simulink model "Unit_Test_Debug_Control"  (R2018b)
settings: Solver=FixedStepDiscrete  StartTime=0.0  StopTime=10.0  FixedStep=fswParams.sample_time_s  RelTol=1e-3
undefined symbols (not defined in the file): fswParams, Mekf_joseph, Mekf_joseph_Lib
libraries: aerolibutil x6, sharedutil x4, dspmtrx3 x2, extended_kalman_filter_lib x1, MEKF_lib x1, satelliteDynamics_lib x1
settings Model: Creator=kashton6  LastModifiedBy=kashton6
settings DataIOCC: ReturnWorkspaceOutputs=on

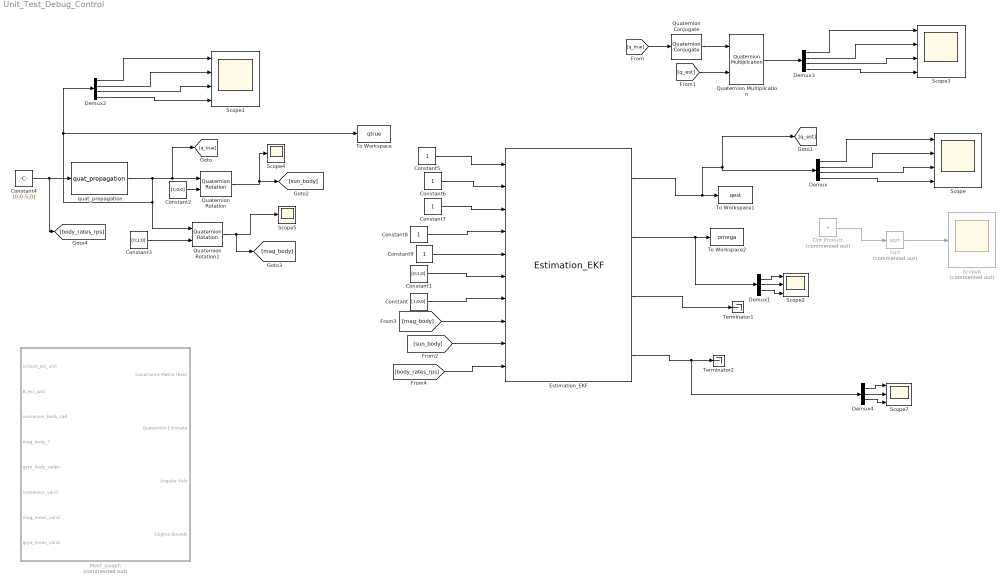
== system Unit_Test_Debug_Control ==
  Constant : Constant  Value=[1;0;0]  VectorParams1D=off
  Constant1 : Constant  Value=[0;1;0]  VectorParams1D=off
  Constant2 : Constant  Value=[1;0;0]  VectorParams1D=off
  Constant3 : Constant  Value=[0;1;0]  VectorParams1D=off
  Constant4 : Constant  Value=[0;0.5;0]  VectorParams1D=off
  Constant{5..9} (5 alike) : Constant
  Demux : Demux
  Demux1 : Demux  Outputs=3
  Demux2 : Demux
  Demux3 : Demux
  Demux4 : Demux  Outputs=3
  Dot Product : DotProduct  Commented=on  InputSameDT=on  OutDataTypeStr=Inherit: Inherit via internal rule
  "Estimation_EKF " : extended_kalman_filter_lib/Estimation_EKF   SystemSampleTime=-1
      link override " ": InitialCondition=fswParams.ekf.ic.rt_valid_gyro
      link override " 1": InitialCondition=fswParams.ekf.ic.rt_valid_mag
      link override " 10": InitialCondition=fswParams.ekf.ic.rt_meas_cov
      link override " 11": InitialCondition=fswParams.ekf.ic.rt_sun_eci_est
      link override " 2": InitialCondition=fswParams.ekf.ic.rt_valid_sun
      link override " 3": InitialCondition=fswParams.ekf.ic.rt_w_body_radps
      link override " 4": InitialCondition=fswParams.ekf.ic.rt_mag_body
      link override " 5": InitialCondition=fswParams.ekf.ic.rt_mag_eci_est
      link override " 6": InitialCondition=fswParams.ekf.ic.rt_sun_body
      link override " 7": InitialCondition=fswParams.ekf.ic.rt_mt_power_ok
      link override " 8": InitialCondition=fswParams.ekf.ic.rt_sc_in_sun
      link override Constant1: Value=fswParams.ekf.meas_cov
      link override Propagate Step /Constant3: Value=fswParams.ekf.proc_cov
      link override Propagate Step /G: Value=fswParams.ekf.G
  Mekf_joseph : Subsystem  Commented=on  AncestorBlock=Mekf_joseph/Mekf_joseph_Lib
  Quaternion Conjugate : aerolibutil/Quaternion Conjugate
      settings: SourceProductName=Aerospace Blockset  SourceProductBaseCode=AE
  Quaternion Multiplication : aerolibutil/Quaternion Multiplication
  Quaternion Rotation : aerolibutil/Quaternion Rotation
  Quaternion Rotation1 : aerolibutil/Quaternion Rotation
  Scope : Scope  NumInputPorts=4
  Scope1 : Scope  NumInputPorts=4
  Scope2 : Scope  NumInputPorts=3
  Scope3 : Scope  NumInputPorts=4
  Scope4 : Scope
  Scope5 : Scope
  Scope6 : Scope  Commented=on
  Scope7 : Scope  NumInputPorts=3
  Sqrt : Sqrt  Commented=on  SaturateOnIntegerOverflow=on
  Terminator1 : Terminator
  Terminator2 : Terminator
  To Workspace : ToWorkspace  VariableName=qtrue  SaveFormat=Timeseries  SampleTime=-1
  To Workspace1 : ToWorkspace  VariableName=qest  SaveFormat=Timeseries  SampleTime=-1
  To Workspace2 : ToWorkspace  VariableName=omega  SaveFormat=Timeseries  SampleTime=-1
  quat_propagation : satelliteDynamics_lib/satelliteDynamics_lib/quat_propagation  SystemSampleTime=-1
  wires:
  Demux3/4 -> Scope3/4
  Sqrt/1 -> Scope6/1
  [q_est] -> Quaternion Multiplication/2
  Dot Product/1 -> Sqrt/1
  Demux3/3 -> Scope3/3
  Demux2/4 -> Scope1/4
  Quaternion Rotation1/1 -> [mag_body], Scope5/1
  Demux3/2 -> Scope3/2
  [q_true] -> Quaternion Conjugate/1
  Demux2/1 -> Scope1/1
  Constant3/1 -> Quaternion Rotation1/2
  Quaternion Multiplication/1 -> Demux3/1
  quat_propagation/1 -> Demux2/1, To Workspace/1, Quaternion Rotation1/1, [q_true], Quaternion Rotation/1
  Demux2/3 -> Scope1/3
  Constant4/1 -> [body_rates_rps], quat_propagation/1
  Constant2/1 -> Quaternion Rotation/2
  Demux1/1 -> Scope2/1
  Demux1/2 -> Scope2/2
  Demux1/3 -> Scope2/3
  Demux3/1 -> Scope3/1
  Demux/3 -> Scope/3
  Quaternion Rotation/1 -> [sun_body], Scope4/1
  Demux/4 -> Scope/4
  Demux/2 -> Scope/2
  Demux/1 -> Scope/1
  Quaternion Conjugate/1 -> Quaternion Multiplication/1
  Demux2/2 -> Scope1/2
  Constant/1 -> "Estimation_EKF "/7
  Constant1/1 -> "Estimation_EKF "/6
  [sun_body] -> "Estimation_EKF "/9
  [mag_body] -> "Estimation_EKF "/8
  [body_rates_rps] -> "Estimation_EKF "/10
  Constant5/1 -> "Estimation_EKF "/1
  Constant6/1 -> "Estimation_EKF "/2
  Constant7/1 -> "Estimation_EKF "/3
  Constant8/1 -> "Estimation_EKF "/4
  Constant9/1 -> "Estimation_EKF "/5
  "Estimation_EKF "/1 -> [q_est], Demux/1, To Workspace1/1
  "Estimation_EKF "/2 -> Demux1/1, To Workspace2/1
  "Estimation_EKF "/3 -> Terminator1/1
  Demux4/3 -> Scope7/3
  "Estimation_EKF "/4 -> Demux4/1, Terminator2/1
  Demux4/2 -> Scope7/2
  Demux4/1 -> Scope7/1

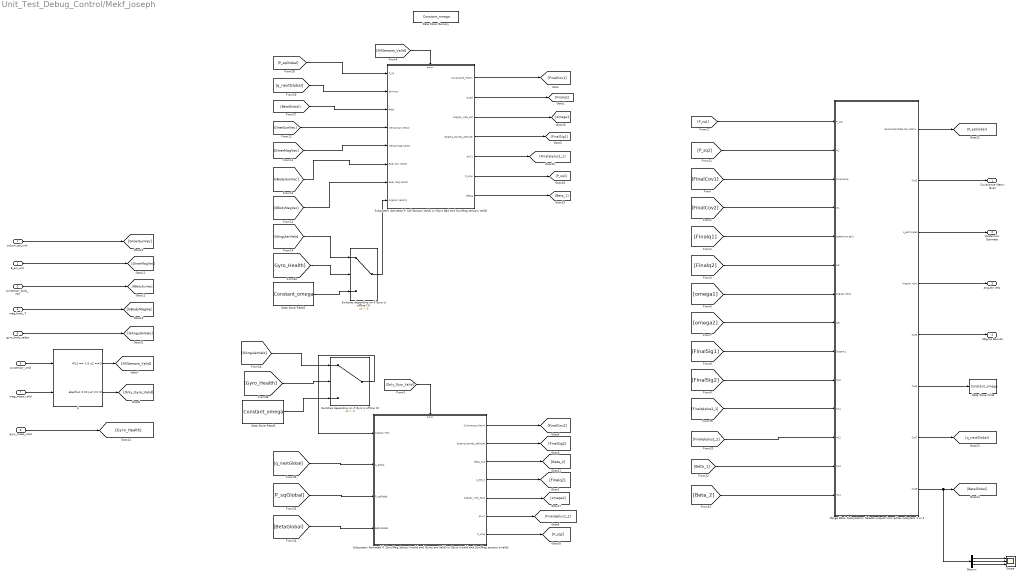
== system Unit_Test_Debug_Control/Mekf_joseph ==
  sc2sun_eci_unit : Inport
  B_eci_unit : Inport  Port=2
  sunsensor_body_rad : Inport  Port=3
  mag_body_T : Inport  Port=4
  gyro_body_radps : Inport  Port=5
  sunsensor_valid : Inport  Port=6
  mag_meas_valid : Inport  Port=7
  gryo_meas_valid : Inport  Port=8
  Data Store Memory : DataStoreMemory  DataStoreName=Constant_omega  ReadBeforeWriteMsg=warning  WriteAfterWriteMsg=warning  WriteAfterReadMsg=warning  InitialValue=fswParams.estimation.ic.w_init  VectorParams1D=off  ShowAdditionalParam=off
  Data Store Read2 : DataStoreRead  DataStoreName=Constant_omega
  Data Store Read3 : DataStoreRead  DataStoreName=Constant_omega
  Data Store Write : DataStoreWrite  DataStoreName=Constant_omega
  Demux : Demux  Outputs=3
  If : If  NumInputs=2  IfExpression=u1 == 1 & u2 ==1  ElseIfExpressions=u1 ==0 |u2 == 0  ShowElse=off
  "Merge Block Subsystems, Selects outputs from either subsytem 1 or 2" : Subsystem
  Scope : Scope  NumInputPorts=3
  Subsystem Activated if: [All Sensors Valid] or [Gyro Bad and Sun/Mag sensors Valid] : Subsystem  TreatAsAtomicUnit=on
  Subsystem Activated if: [Sun/Mag Sensor Invalid and Gyros are Valid] or [Gyro Invalid and Sun/Mag sensors Invalid] : Subsystem  TreatAsAtomicUnit=on
  Switches depending on if Gyro is offline (1) : Switch  Criteria=u2 > Threshold
  Switches depending on if Gyro is offline (2) : Switch  Criteria=u2 > Threshold
  Covariance Matrix (6x6) : Outport
  "Quaternion Estimate " : Outport  Port=2
  "Angular Velo " : Outport  Port=3
  "3Sigma Bounds " : Outport  Port=4
  wires:
  Subsystem Activated if: [Sun/Mag Sensor Invalid and Gyros are Valid] or [Gyro Invalid and Sun/Mag sensors Invalid]/6(qk+1) -> [Finalqkplus1_2]
  Switches depending on if Gyro is offline (2)/1 -> Subsystem Activated if: [Sun/Mag Sensor Invalid and Gyros are Valid] or [Gyro Invalid and Sun/Mag sensors Invalid]/1(Angular Velo)
  Switches depending on if Gyro is offline (1)/1 -> Subsystem Activated if: [All Sensors Valid] or [Gyro Bad and Sun/Mag sensors Valid]/8(Angular Velocity)
  [GAngularVelo] -> Switches depending on if Gyro is offline (1)/1
  [GAngularVelo] -> Switches depending on if Gyro is offline (2)/1
  [GBodySunVec] -> Subsystem Activated if: [All Sensors Valid] or [Gyro Bad and Sun/Mag sensors Valid]/6(Body Sun Vector)
  [GInerMagVec] -> Subsystem Activated if: [All Sensors Valid] or [Gyro Bad and Sun/Mag sensors Valid]/5(Inertial Mag Vector)
  [GBodyMagVec] -> Subsystem Activated if: [All Sensors Valid] or [Gyro Bad and Sun/Mag sensors Valid]/7(Body Mag Vector)
  Subsystem Activated if: [All Sensors Valid] or [Gyro Bad and Sun/Mag sensors Valid]/2(q_est) -> [Finalq1]
  Subsystem Activated if: [All Sensors Valid] or [Gyro Bad and Sun/Mag sensors Valid]/1(Covariance_Matrix) -> [FinalCov1]
  [Only_Gyro_Valid] -> Subsystem Activated if: [Sun/Mag Sensor Invalid and Gyros are Valid] or [Gyro Invalid and Sun/Mag sensors Invalid]/Action
  Subsystem Activated if: [All Sensors Valid] or [Gyro Bad and Sun/Mag sensors Valid]/4(3sigma_bounds_attitude) -> [FinalSig1]
  Subsystem Activated if: [Sun/Mag Sensor Invalid and Gyros are Valid] or [Gyro Invalid and Sun/Mag sensors Invalid]/4(q_est_k) -> [Finalq2]
  [GInerSunVec] -> Subsystem Activated if: [All Sensors Valid] or [Gyro Bad and Sun/Mag sensors Valid]/4(Inertial Sun Vector)
  Subsystem Activated if: [Sun/Mag Sensor Invalid and Gyros are Valid] or [Gyro Invalid and Sun/Mag sensors Invalid]/1(Covariance_Matrix) -> [FinalCov2]
  [AllSensors_Valid] -> Subsystem Activated if: [All Sensors Valid] or [Gyro Bad and Sun/Mag sensors Valid]/Action
  Subsystem Activated if: [Sun/Mag Sensor Invalid and Gyros are Valid] or [Gyro Invalid and Sun/Mag sensors Invalid]/2(3sigma_bounds_attitude) -> [FinalSig2]
  [q_nextGlobal] -> Subsystem Activated if: [Sun/Mag Sensor Invalid and Gyros are Valid] or [Gyro Invalid and Sun/Mag sensors Invalid]/2(q_global)
  Subsystem Activated if: [All Sensors Valid] or [Gyro Bad and Sun/Mag sensors Valid]/5(qk+1) -> [Finalqkplus1_1]
  [P_sqGlobal] -> Subsystem Activated if: [Sun/Mag Sensor Invalid and Gyros are Valid] or [Gyro Invalid and Sun/Mag sensors Invalid]/3(P_sqGlobal)
  [BetaGlobal] -> Subsystem Activated if: [Sun/Mag Sensor Invalid and Gyros are Valid] or [Gyro Invalid and Sun/Mag sensors Invalid]/4(Beta Global)
  [BetaGlobal] -> Subsystem Activated if: [All Sensors Valid] or [Gyro Bad and Sun/Mag sensors Valid]/3(Beta)
  Subsystem Activated if: [All Sensors Valid] or [Gyro Bad and Sun/Mag sensors Valid]/3(Angular_Velo_est) -> [omega1]
  Subsystem Activated if: [All Sensors Valid] or [Gyro Bad and Sun/Mag sensors Valid]/6("P_prop ") -> [P_sq1]
  Subsystem Activated if: [All Sensors Valid] or [Gyro Bad and Sun/Mag sensors Valid]/7(Betaa) -> [Beta_1]
  Subsystem Activated if: [Sun/Mag Sensor Invalid and Gyros are Valid] or [Gyro Invalid and Sun/Mag sensors Invalid]/7("P_prop ") -> [P_sq2]
  Subsystem Activated if: [Sun/Mag Sensor Invalid and Gyros are Valid] or [Gyro Invalid and Sun/Mag sensors Invalid]/3(Beta_Out) -> [Beta_2]
  Subsystem Activated if: [Sun/Mag Sensor Invalid and Gyros are Valid] or [Gyro Invalid and Sun/Mag sensors Invalid]/5(Angular_Velo_est1) -> [omega2]
  [q_nextGlobal] -> Subsystem Activated if: [All Sensors Valid] or [Gyro Bad and Sun/Mag sensors Valid]/2(qkminus)
  [P_sqGlobal] -> Subsystem Activated if: [All Sensors Valid] or [Gyro Bad and Sun/Mag sensors Valid]/1(P_sq)
  If/1 -> [AllSensors_Valid]
  If/2 -> [Only_Gyro_Valid]
  [Gyro_Health] -> Switches depending on if Gyro is offline (1)/2
  Data Store Read2/1 -> Switches depending on if Gyro is offline (1)/3
  [Gyro_Health] -> Switches depending on if Gyro is offline (2)/2
  Data Store Read3/1 -> Switches depending on if Gyro is offline (2)/3
  [P_sq1] -> "Merge Block Subsystems, Selects outputs from either subsytem 1 or 2"/1(P_sq1)
  [P_sq2] -> "Merge Block Subsystems, Selects outputs from either subsytem 1 or 2"/2(In2)
  [FinalCov1] -> "Merge Block Subsystems, Selects outputs from either subsytem 1 or 2"/3(covariance)
  [FinalCov2] -> "Merge Block Subsystems, Selects outputs from either subsytem 1 or 2"/4(In4)
  [Finalq1] -> "Merge Block Subsystems, Selects outputs from either subsytem 1 or 2"/5(quaternion est1)
  [Finalq2] -> "Merge Block Subsystems, Selects outputs from either subsytem 1 or 2"/6(In6)
  [omega1] -> "Merge Block Subsystems, Selects outputs from either subsytem 1 or 2"/7(angular velo1)
  [omega2] -> "Merge Block Subsystems, Selects outputs from either subsytem 1 or 2"/8(In8)
  [FinalSig1] -> "Merge Block Subsystems, Selects outputs from either subsytem 1 or 2"/9(3sigma 1)
  [FinalSig2] -> "Merge Block Subsystems, Selects outputs from either subsytem 1 or 2"/10(In10)
  [Finalqkplus1_1] -> "Merge Block Subsystems, Selects outputs from either subsytem 1 or 2"/11(In11)
  [Finalqkplus1_2] -> "Merge Block Subsystems, Selects outputs from either subsytem 1 or 2"/12(In12)
  [Beta_1] -> "Merge Block Subsystems, Selects outputs from either subsytem 1 or 2"/13(In13)
  [Beta_2] -> "Merge Block Subsystems, Selects outputs from either subsytem 1 or 2"/14(In14)
  "Merge Block Subsystems, Selects outputs from either subsytem 1 or 2"/1(Squre Root State Cov Matrix) -> [P_sqGlobal]
  "Merge Block Subsystems, Selects outputs from either subsytem 1 or 2"/2(Out2) -> Covariance Matrix (6x6)/1
  "Merge Block Subsystems, Selects outputs from either subsytem 1 or 2"/3(q_estimated) -> "Quaternion Estimate "/1
  "Merge Block Subsystems, Selects outputs from either subsytem 1 or 2"/4(Angular Velo) -> "Angular Velo "/1
  "Merge Block Subsystems, Selects outputs from either subsytem 1 or 2"/6(Out5) -> Data Store Write/1
  "Merge Block Subsystems, Selects outputs from either subsytem 1 or 2"/5(Out6) -> "3Sigma Bounds "/1
  "Merge Block Subsystems, Selects outputs from either subsytem 1 or 2"/7(Out7) -> [q_nextGlobal]
  sc2sun_eci_unit/1 -> [GInerSunVec]
  sunsensor_body_rad/1 -> [GBodySunVec]
  sunsensor_valid/1 -> If/1
  mag_meas_valid/1 -> If/2
  gryo_meas_valid/1 -> [Gyro_Health]
  B_eci_unit/1 -> [GInerMagVec]
  mag_body_T/1 -> [GBodyMagVec]
  gyro_body_radps/1 -> [GAngularVelo]
  Demux/3 -> Scope/3
  Demux/2 -> Scope/2
  "Merge Block Subsystems, Selects outputs from either subsytem 1 or 2"/8(Out8) -> Demux/1, [BetaGlobal]
  Demux/1 -> Scope/1

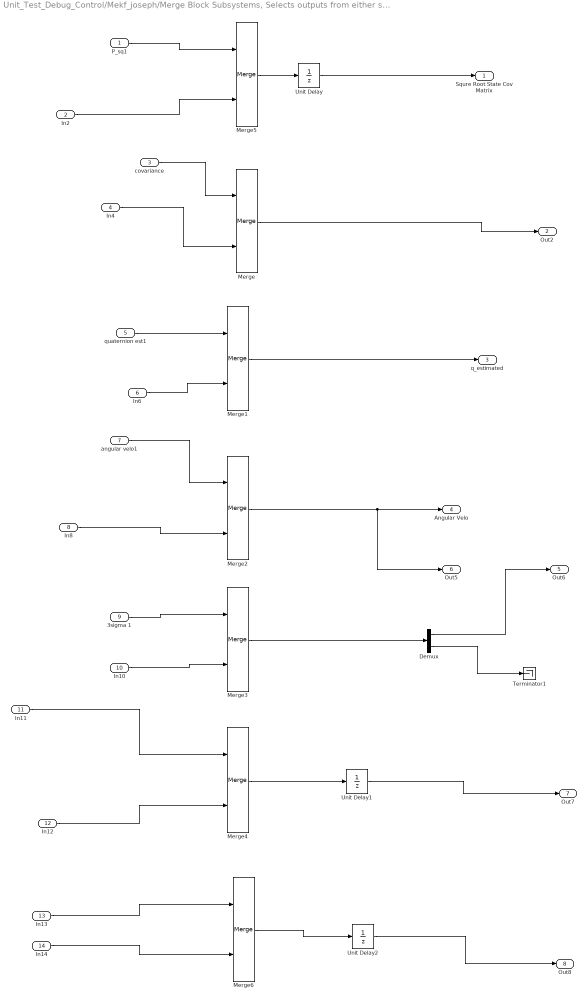
== system Unit_Test_Debug_Control/Mekf_joseph/Merge Block Subsystems, Selects outputs from either subsytem 1 or 2 ==
  P_sq1 : Inport
  In2 : Inport  Port=2
  covariance : Inport  Port=3
  In4 : Inport  Port=4
  quaternion est1 : Inport  Port=5
  In6 : Inport  Port=6
  angular velo1 : Inport  Port=7
  In8 : Inport  Port=8
  3sigma 1 : Inport  Port=9
  In10 : Inport  Port=10
  In11 : Inport  Port=11
  In12 : Inport  Port=12
  In13 : Inport  Port=13
  In14 : Inport  Port=14
  Demux : Demux  Outputs=2
  Merge{,1..6} (7 alike) : Merge
  Terminator1 : Terminator
  Unit Delay : UnitDelay  InitialCondition=fswParams.estimation.ic.P_init  SampleTime=-1  HasFrameUpgradeWarning=on
  Unit Delay1 : UnitDelay  InitialCondition=fswParams.estimation.ic.quat_est_init  SampleTime=-1  HasFrameUpgradeWarning=on
  Unit Delay2 : UnitDelay  InitialCondition=fswParams.estimation.ic.Beta_init  SampleTime=-1  HasFrameUpgradeWarning=on
  Squre Root State Cov Matrix : Outport
  Out2 : Outport  Port=2
  q_estimated : Outport  Port=3
  Angular Velo : Outport  Port=4
  Out6 : Outport  Port=5
  Out5 : Outport  Port=6
  Out7 : Outport  Port=7
  Out8 : Outport  Port=8
  wires:
  Merge3/1 -> Demux/1
  Merge2/1 -> Out5/1, Angular Velo/1
  Unit Delay1/1 -> Out7/1
  Demux/2 -> Terminator1/1
  Merge6/1 -> Unit Delay2/1
  3sigma 1/1 -> Merge3/1
  quaternion est1/1 -> Merge1/1
  In14/1 -> Merge6/2
  angular velo1/1 -> Merge2/1
  In11/1 -> Merge4/1
  Merge5/1 -> Unit Delay/1
  In10/1 -> Merge3/2
  In2/1 -> Merge5/2
  covariance/1 -> Merge/1
  Merge4/1 -> Unit Delay1/1
  In4/1 -> Merge/2
  Demux/1 -> Out6/1
  In13/1 -> Merge6/1
  Merge/1 -> Out2/1
  In6/1 -> Merge1/2
  In8/1 -> Merge2/2
  In12/1 -> Merge4/2
  P_sq1/1 -> Merge5/1
  Unit Delay2/1 -> Out8/1
  Unit Delay/1 -> Squre Root State Cov Matrix/1
  Merge1/1 -> q_estimated/1

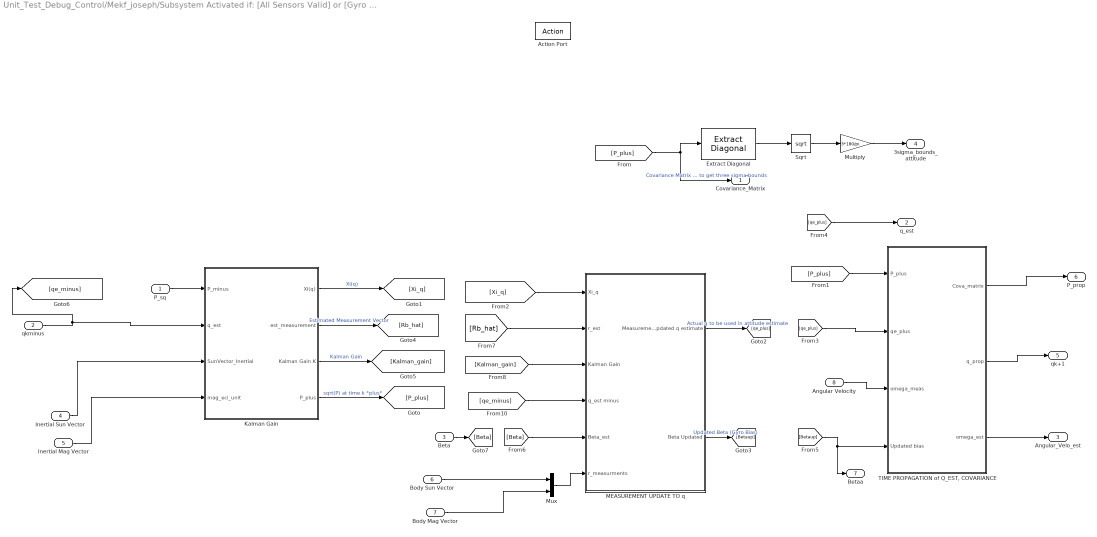
== system Unit_Test_Debug_Control/Mekf_joseph/Subsystem Activated if: [All Sensors Valid] or [Gyro Bad and Sun//Mag sensors Valid] ==
  P_sq : Inport
  qkminus : Inport  Port=2
  Beta : Inport  Port=3
  Inertial Sun Vector : Inport  Port=4
  Inertial Mag Vector : Inport  Port=5
  Body Sun Vector : Inport  Port=6
  Body Mag Vector : Inport  Port=7
  Angular Velocity : Inport  Port=8
  Action Port : ActionPort
  Extract Diagonal : dspmtrx3/Extract Diagonal
      settings: SourceProductName=DSP System Toolbox  SourceProductBaseCode=DS
  Kalman Gain : Subsystem  AncestorBlock=MEKF_LibraryR2018b/Multiplicative Extended Kalman Filter/Kalman Gain
  "MEASUREMENT UPDATE TO q " : Subsystem  AncestorBlock=MEKF_LibraryR2018b/Multiplicative Extended Kalman Filter/MEASUREMENT UPDATE TO q AND COVARIANCE2
  Multiply : Gain  Gain=3*180/pi
  Mux : Mux  Inputs=2
  Sqrt : Sqrt  SaturateOnIntegerOverflow=on
  "TIME PROPAGATION of Q_EST, COVARIANCE" : Subsystem  AncestorBlock=MEKF_Library/Multiplicative Extended Kalman Filter/TIME PROPAGATION of Q_EST, COVARIANCE
  Covariance_Matrix : Outport
  q_est : Outport  Port=2
  Angular_Velo_est : Outport  Port=3
  3sigma_bounds_attitude : Outport  Port=4
  qk+1 : Outport  Port=5
  "P_prop " : Outport  Port=6
  Betaa : Outport  Port=7
  wires:
  Inertial Sun Vector/1 -> Kalman Gain/3(SunVector_Inertial)
  [qe_plus] -> q_est/1
  "TIME PROPAGATION of Q_EST, COVARIANCE"/2(q_prop) -> qk+1/1
  "TIME PROPAGATION of Q_EST, COVARIANCE"/3(omega_est) -> Angular_Velo_est/1
  [P_plus] -> Extract Diagonal/1, Covariance_Matrix/1  "Covariance Matrix from which to get three sigma bounds"
  qkminus/1 -> [qe_minus], Kalman Gain/2(q_est)
  Extract Diagonal/1 -> Sqrt/1
  Angular Velocity/1 -> "TIME PROPAGATION of Q_EST, COVARIANCE"/3(omega_meas)
  P_sq/1 -> Kalman Gain/1(P_minus)
  [qe_plus] -> "TIME PROPAGATION of Q_EST, COVARIANCE"/2(qe_plus)
  "MEASUREMENT UPDATE TO q "/2(Beta Updated) -> [Betaup]  "Updated Beta (Gyro Bias)"
  [Rb_hat] -> "MEASUREMENT UPDATE TO q "/2(r_est)
  "TIME PROPAGATION of Q_EST, COVARIANCE"/1(Cova_matrix) -> "P_prop "/1
  Kalman Gain/4(P_plus) -> [P_plus]  "sqrt(P) at time k *plus*"
  Kalman Gain/3(Kalman Gain K) -> [Kalman_gain]  "Kalman Gain"
  [qe_minus] -> "MEASUREMENT UPDATE TO q "/4(q_est minus)
  Kalman Gain/1(Xi(q)) -> [Xi_q]  "Xi(q)"
  Sqrt/1 -> Multiply/1
  [Betaup] -> "TIME PROPAGATION of Q_EST, COVARIANCE"/4(Updated bias), Betaa/1
  [Beta] -> "MEASUREMENT UPDATE TO q "/5(Beta_est)
  "MEASUREMENT UPDATE TO q "/1(Measurement updated q estimate) -> [qe_plus]  "Actual q to be used in attitude estimate"
  [P_plus] -> "TIME PROPAGATION of Q_EST, COVARIANCE"/1(P_plus)
  Kalman Gain/2(est_measurement) -> [Rb_hat]  "Estimated Measurement Vector"
  [Xi_q] -> "MEASUREMENT UPDATE TO q "/1(Xi_q)
  [Kalman_gain] -> "MEASUREMENT UPDATE TO q "/3(Kalman Gain)
  Inertial Mag Vector/1 -> Kalman Gain/4("mag_eci_unit ")
  Body Sun Vector/1 -> Mux/1
  Body Mag Vector/1 -> Mux/2
  Mux/1 -> "MEASUREMENT UPDATE TO q "/6(r_measurments)
  Multiply/1 -> 3sigma_bounds_attitude/1
  Beta/1 -> [Beta]

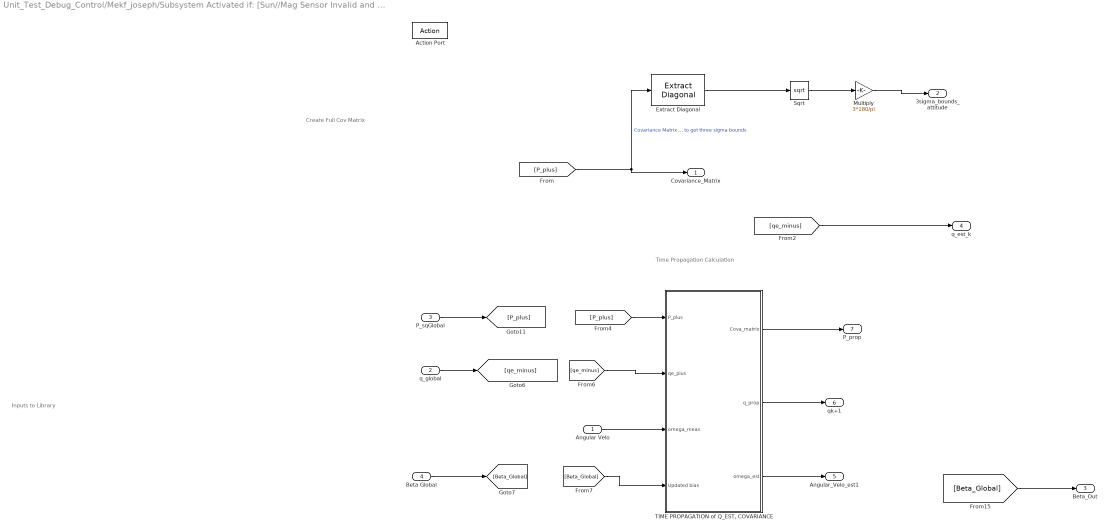
== system Unit_Test_Debug_Control/Mekf_joseph/Subsystem Activated if: [Sun//Mag Sensor Invalid and Gyros are Valid] or [Gyro Invalid and Sun//Mag sensors Invalid] ==
  note: Time Propagation Calculation
  note: Inputs to Library
  note: Create Full Cov Matrix
  Angular Velo : Inport
  q_global : Inport  Port=2
  P_sqGlobal : Inport  Port=3
  Beta Global : Inport  Port=4
  Action Port : ActionPort
  Extract Diagonal : dspmtrx3/Extract Diagonal
      settings: SourceProductName=DSP System Toolbox  SourceProductBaseCode=DS
  Multiply : Gain  Gain=3*180/pi
  Sqrt : Sqrt  SaturateOnIntegerOverflow=on
  "TIME PROPAGATION of Q_EST, COVARIANCE" : Subsystem  AncestorBlock=|
      | Mekf_joseph/Mekf_joseph_Lib/Subsystem Activated if: [All Sensors Valid]
      | or
      | [Gyro Bad and Sun//Mag sensors Valid]/TIME PROPAGATION of Q_EST, COVARIANCE
  Covariance_Matrix : Outport
  3sigma_bounds_attitude : Outport  Port=2
  Beta_Out : Outport  Port=3
  q_est_k : Outport  Port=4
  Angular_Velo_est1 : Outport  Port=5
  qk+1 : Outport  Port=6
  "P_prop " : Outport  Port=7
  wires:
  [P_plus] -> "TIME PROPAGATION of Q_EST, COVARIANCE"/1(P_plus)
  "TIME PROPAGATION of Q_EST, COVARIANCE"/2(q_prop) -> qk+1/1
  "TIME PROPAGATION of Q_EST, COVARIANCE"/1(Cova_matrix) -> "P_prop "/1
  [Beta_Global] -> "TIME PROPAGATION of Q_EST, COVARIANCE"/4(Updated bias)
  "TIME PROPAGATION of Q_EST, COVARIANCE"/3(omega_est) -> Angular_Velo_est1/1
  Angular Velo/1 -> "TIME PROPAGATION of Q_EST, COVARIANCE"/3(omega_meas)
  [qe_minus] -> "TIME PROPAGATION of Q_EST, COVARIANCE"/2(qe_plus)
  q_global/1 -> [qe_minus]
  Beta Global/1 -> [Beta_Global]
  Extract Diagonal/1 -> Sqrt/1
  P_sqGlobal/1 -> [P_plus]
  [qe_minus] -> q_est_k/1
  [P_plus] -> Extract Diagonal/1, Covariance_Matrix/1  "Covariance Matrix from which to get three sigma bounds"
  [Beta_Global] -> Beta_Out/1
  Multiply/1 -> 3sigma_bounds_attitude/1
  Sqrt/1 -> Multiply/1

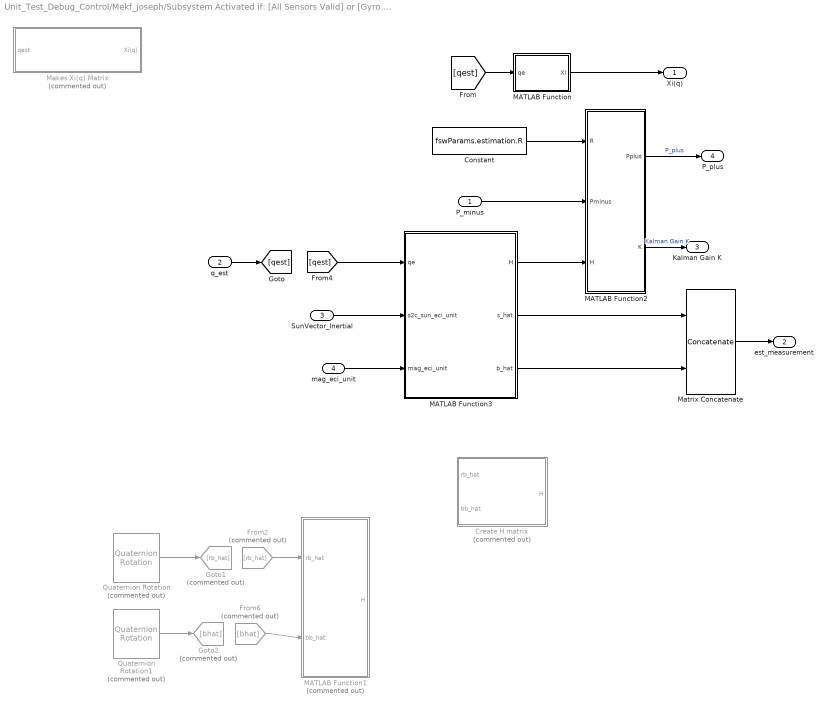
== system Unit_Test_Debug_Control/Mekf_joseph/Subsystem Activated if: [All Sensors Valid] or [Gyro Bad and Sun//Mag sensors Valid]/Kalman Gain ==
  P_minus : Inport
  q_est : Inport  Port=2
  SunVector_Inertial : Inport  Port=3
  "mag_eci_unit " : Inport  Port=4
  Constant : Constant  Value=fswParams.estimation.R  VectorParams1D=off
  Create H matrix : Subsystem  Commented=on
  From2 : From  Commented=on  GotoTag=rb_hat
  From6 : From  Commented=on  GotoTag=bhat
  Goto1 : Goto  Commented=on  GotoTag=rb_hat
  Goto2 : Goto  Commented=on  GotoTag=bhat
  MATLAB Function : MATLAB Function  TreatAsAtomicUnit=on
  MATLAB Function1 : MATLAB Function  Commented=on  TreatAsAtomicUnit=on
  MATLAB Function2 : MATLAB Function  TreatAsAtomicUnit=on
  MATLAB Function3 : MATLAB Function  TreatAsAtomicUnit=on
  Makes Xi(q) Matrix : Subsystem  Commented=on
  Matrix Concatenate : Concatenate  Mode=Multidimensional array
  Quaternion Rotation : aerolibutil/Quaternion Rotation  Commented=on
  Quaternion Rotation1 : aerolibutil/Quaternion Rotation  Commented=on
  Xi(q) : Outport
  est_measurement : Outport  Port=2
  Kalman Gain K : Outport  Port=3
  P_plus : Outport  Port=4
  wires:
  MATLAB Function3/1(H) -> MATLAB Function2/3(H)
  "mag_eci_unit "/1 -> MATLAB Function3/3(mag_eci_unit)
  SunVector_Inertial/1 -> MATLAB Function3/2(s2c_sun_eci_unit)
  [qest] -> MATLAB Function3/1(qe)
  From6/1 -> MATLAB Function1/2(bb_hat)
  From2/1 -> MATLAB Function1/1(rb_hat)
  P_minus/1 -> MATLAB Function2/2(Pminus)
  MATLAB Function2/2(K) -> Kalman Gain K/1  "Kalman Gain K"
  MATLAB Function2/1(Pplus) -> P_plus/1  "P_plus"
  q_est/1 -> [qest]
  Quaternion Rotation/1 -> Goto1/1
  Quaternion Rotation1/1 -> Goto2/1
  MATLAB Function3/2(s_hat) -> Matrix Concatenate/1
  MATLAB Function3/3(b_hat) -> Matrix Concatenate/2
  Matrix Concatenate/1 -> est_measurement/1
  Constant/1 -> MATLAB Function2/1(R)
  [qest] -> MATLAB Function/1(qe)
  MATLAB Function/1(XI) -> Xi(q)/1

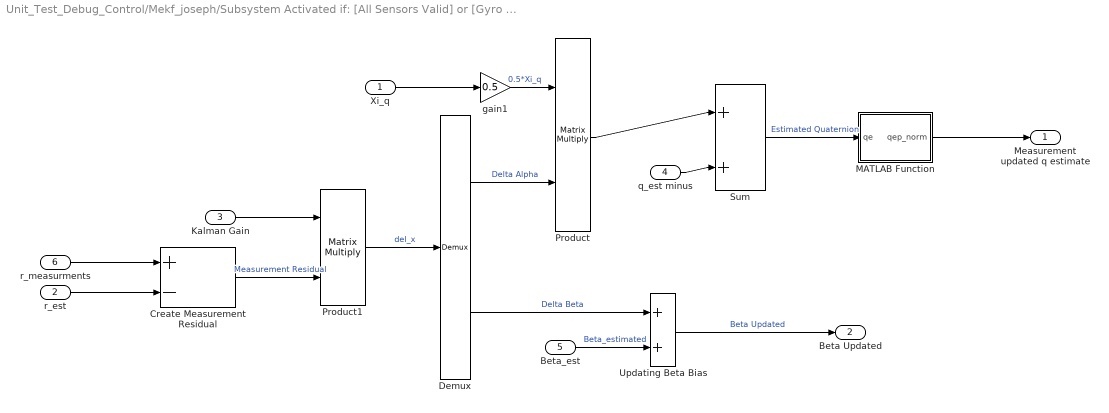
== system Unit_Test_Debug_Control/Mekf_joseph/Subsystem Activated if: [All Sensors Valid] or [Gyro Bad and Sun//Mag sensors Valid]/MEASUREMENT UPDATE TO q  ==
  Xi_q : Inport
  r_est : Inport  Port=2
  Kalman Gain : Inport  Port=3
  q_est minus : Inport  Port=4
  Beta_est : Inport  Port=5
  r_measurments : Inport  Port=6
  Create Measurement Residual : Sum  Inputs=+-
  Demux : Demux  Outputs=[3;3]
  MATLAB Function : MATLAB Function  TreatAsAtomicUnit=on
  Product : Product  Inputs=**  Multiplication=Matrix(*)
  Product1 : Product  Multiplication=Matrix(*)
  Sum : Sum  Inputs=|++
  "Updating Beta Bias " : Sum
  gain1 : Gain  Gain=0.5
  Measurement updated q estimate : Outport
  Beta Updated : Outport  Port=2
  wires:
  Demux/1 -> Product/2  "Delta Alpha"
  gain1/1 -> Product/1  "0.5*Xi_q"
  Demux/2 -> "Updating Beta Bias "/1  "Delta Beta"
  Product/1 -> Sum/1
  Product1/1 -> Demux/1  "del_x"
  r_est/1 -> Create Measurement Residual/2
  Create Measurement Residual/1 -> Product1/2  "Measurement Residual"
  "Updating Beta Bias "/1 -> Beta Updated/1  "Beta Updated"
  Beta_est/1 -> "Updating Beta Bias "/2  "Beta_estimated"
  q_est minus/1 -> Sum/2
  Kalman Gain/1 -> Product1/1
  r_measurments/1 -> Create Measurement Residual/1
  Xi_q/1 -> gain1/1
  Sum/1 -> MATLAB Function/1(qe)  "Estimated Quaternion"
  MATLAB Function/1(qep_norm) -> Measurement updated q estimate/1

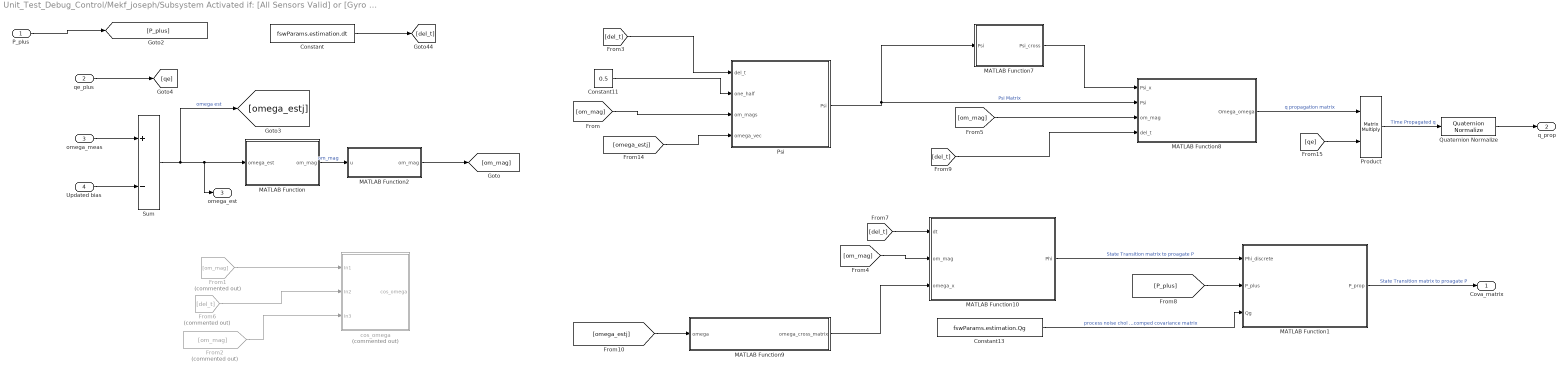
== system Unit_Test_Debug_Control/Mekf_joseph/Subsystem Activated if: [All Sensors Valid] or [Gyro Bad and Sun//Mag sensors Valid]/TIME PROPAGATION of Q_EST, COVARIANCE ==
  P_plus : Inport
  qe_plus : Inport  Port=2
  omega_meas : Inport  Port=3
  Updated bias : Inport  Port=4
  Constant : Constant  Value=fswParams.estimation.dt
  Constant11 : Constant  Value=0.5
  Constant13 : Constant  Value=fswParams.estimation.Qg  VectorParams1D=off
  From1 : From  Commented=on  GotoTag=om_mag
  From2 : From  Commented=on  GotoTag=om_mag
  From6 : From  Commented=on  GotoTag=del_t
  MATLAB Function : MATLAB Function  TreatAsAtomicUnit=on
  MATLAB Function1 : MATLAB Function  TreatAsAtomicUnit=on
  MATLAB Function10 : MATLAB Function  TreatAsAtomicUnit=on
  MATLAB Function2 : MATLAB Function  TreatAsAtomicUnit=on
  MATLAB Function7 : MATLAB Function  TreatAsAtomicUnit=on
  MATLAB Function8 : MATLAB Function  TreatAsAtomicUnit=on
  MATLAB Function9 : MATLAB Function  TreatAsAtomicUnit=on
  Product : Product  Multiplication=Matrix(*)
  Psi : Subsystem
  Quaternion Normalize : sharedutil/Quaternion Normalize  aMode=aMode
      settings: SourceProductName=Aerospace Blockset  SourceProductBaseCode=AE
  Sum : Sum  Inputs=+-
  cos_omega : Subsystem  Commented=on
  Cova_matrix : Outport
  q_prop : Outport  Port=2
  omega_est : Outport  Port=3
  wires:
  Quaternion Normalize/1 -> q_prop/1
  P_plus/1 -> [P_plus]
  qe_plus/1 -> [qe]
  Updated bias/1 -> Sum/2
  omega_meas/1 -> Sum/1
  [del_t] -> MATLAB Function8/4(del_t)
  MATLAB Function7/1(Psi_cross) -> MATLAB Function8/1(Psi_x)
  MATLAB Function8/1(Omega_omega) -> Product/1  "q propagation matrix"
  MATLAB Function9/1(omega_cross_matrix) -> MATLAB Function10/3(omega_x)
  MATLAB Function10/1(Phi) -> MATLAB Function1/1(Phi_discrete)  "State Transition matrix to proagate P"
  Product/1 -> Quaternion Normalize/1  "Time Propagated q"
  Constant13/1 -> MATLAB Function1/3(Qg)  "process noise chol decomped covariance matrix"
  MATLAB Function/1(om_mag) -> MATLAB Function2/1(u)  "om_mag"
  [om_mag] -> MATLAB Function10/2(om_mag)
  [om_mag] -> MATLAB Function8/3(om_mag)
  [del_t] -> MATLAB Function10/1(dt)
  [P_plus] -> MATLAB Function1/2(P_plus)
  [omega_estj] -> MATLAB Function9/1(omega)
  [qe] -> Product/2
  From1/1 -> cos_omega/1(In1)
  From2/1 -> cos_omega/3(In3)
  Psi/1(Psi) -> MATLAB Function8/2(Psi), MATLAB Function7/1(Psi)  "Psi Matrix"
  [del_t] -> Psi/1(del_t)
  Constant11/1 -> Psi/2(one_half)
  [omega_estj] -> Psi/4(omega_vec)
  [om_mag] -> Psi/3(om_mags)
  Sum/1 -> MATLAB Function/1(omega_est), omega_est/1, [omega_estj]  "omega est"
  From6/1 -> cos_omega/2(In2)
  Constant/1 -> [del_t]
  MATLAB Function2/1(om_mag) -> [om_mag]
  MATLAB Function1/1(P_prop) -> Cova_matrix/1  "State Transition matrix to proagate P"

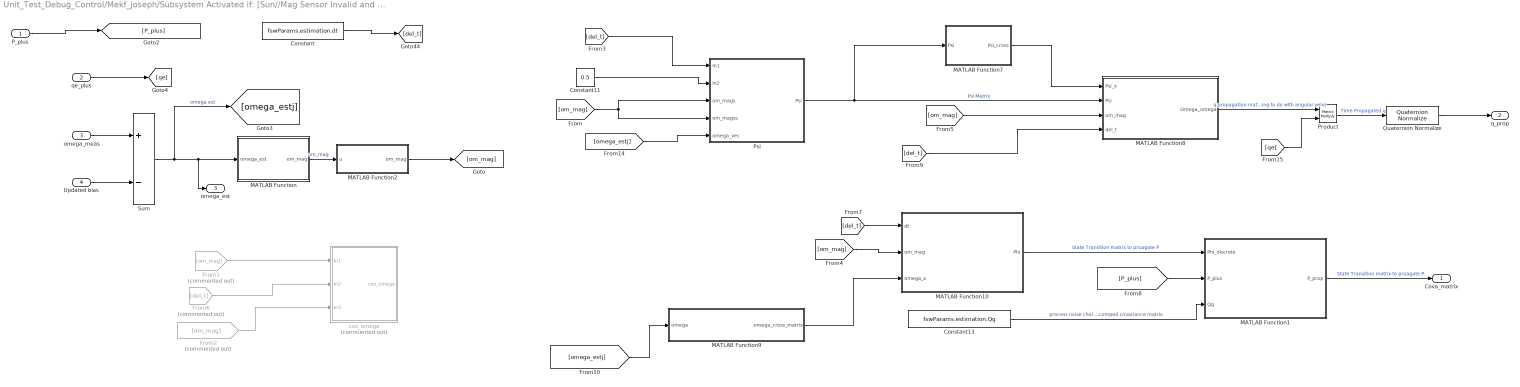
== system Unit_Test_Debug_Control/Mekf_joseph/Subsystem Activated if: [Sun//Mag Sensor Invalid and Gyros are Valid] or [Gyro Invalid and Sun//Mag sensors Invalid]/TIME PROPAGATION of Q_EST, COVARIANCE ==
  P_plus : Inport
  qe_plus : Inport  Port=2
  omega_meas : Inport  Port=3
  Updated bias : Inport  Port=4
  Constant : Constant  Value=fswParams.estimation.dt
  Constant11 : Constant  Value=0.5
  Constant13 : Constant  Value=fswParams.estimation.Qg  VectorParams1D=off
  From1 : From  Commented=on  GotoTag=om_mag
  From2 : From  Commented=on  GotoTag=om_mag
  From6 : From  Commented=on  GotoTag=del_t
  MATLAB Function : MATLAB Function  TreatAsAtomicUnit=on
  MATLAB Function1 : MATLAB Function  TreatAsAtomicUnit=on
  MATLAB Function10 : MATLAB Function  TreatAsAtomicUnit=on
  MATLAB Function2 : MATLAB Function  TreatAsAtomicUnit=on
  MATLAB Function7 : MATLAB Function  TreatAsAtomicUnit=on
  MATLAB Function8 : MATLAB Function  TreatAsAtomicUnit=on
  MATLAB Function9 : MATLAB Function  TreatAsAtomicUnit=on
  Product : Product  Multiplication=Matrix(*)
  Psi : Subsystem
  Quaternion Normalize : sharedutil/Quaternion Normalize  aMode=aMode
      settings: SourceProductName=Aerospace Blockset  SourceProductBaseCode=AE
  Sum : Sum  Inputs=+-
  cos_omega : Subsystem  Commented=on
  Cova_matrix : Outport
  q_prop : Outport  Port=2
  omega_est : Outport  Port=3
  wires:
  Quaternion Normalize/1 -> q_prop/1
  P_plus/1 -> [P_plus]
  qe_plus/1 -> [qe]
  Updated bias/1 -> Sum/2
  omega_meas/1 -> Sum/1
  [del_t] -> MATLAB Function8/4(del_t)
  MATLAB Function7/1(Psi_cross) -> MATLAB Function8/1(Psi_x)
  MATLAB Function8/1(Omega_omega) -> Product/1  "q propagation matrix (nothing to do with angular velo)"
  MATLAB Function9/1(omega_cross_matrix) -> MATLAB Function10/3(omega_x)
  MATLAB Function10/1(Phi) -> MATLAB Function1/1(Phi_discrete)  "State Transition matrix to proagate P"
  Product/1 -> Quaternion Normalize/1  "Time Propagated q"
  Constant13/1 -> MATLAB Function1/3(Qg)  "process noise chol decomped covariance matrix"
  MATLAB Function/1(om_mag) -> MATLAB Function2/1(u)  "om_mag"
  [om_mag] -> MATLAB Function10/2(om_mag)
  [om_mag] -> MATLAB Function8/3(om_mag)
  [del_t] -> MATLAB Function10/1(dt)
  [P_plus] -> MATLAB Function1/2(P_plus)
  [omega_estj] -> MATLAB Function9/1(omega)
  [qe] -> Product/2
  From1/1 -> cos_omega/1(In1)
  From2/1 -> cos_omega/3(In3)
  Psi/1(Psi) -> MATLAB Function8/2(Psi), MATLAB Function7/1(Psi)  "Psi Matrix"
  [del_t] -> Psi/1(In1)
  Constant11/1 -> Psi/2(In2)
  [omega_estj] -> Psi/5(omega_vec)
  [om_mag] -> Psi/3(om_mags), Psi/4(om_magss)
  Sum/1 -> MATLAB Function/1(omega_est), omega_est/1, [omega_estj]  "omega est"
  From6/1 -> cos_omega/2(In2)
  Constant/1 -> [del_t]
  MATLAB Function2/1(om_mag) -> [om_mag]
  MATLAB Function1/1(P_prop) -> Cova_matrix/1  "State Transition matrix to proagate P"

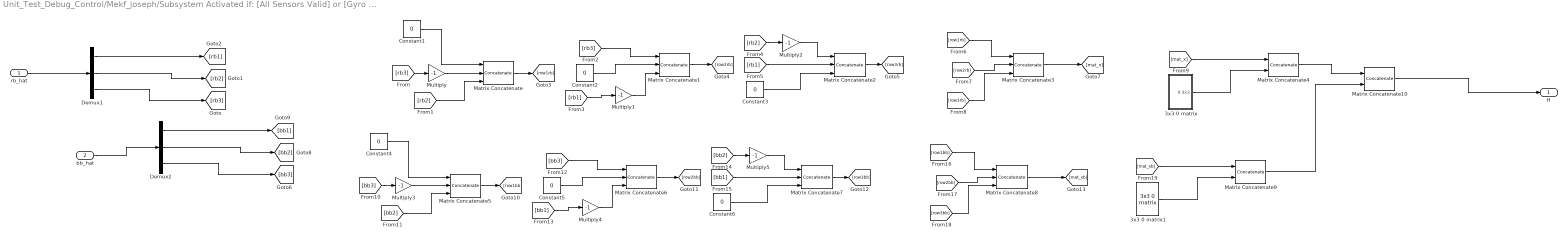
== system Unit_Test_Debug_Control/Mekf_joseph/Subsystem Activated if: [All Sensors Valid] or [Gyro Bad and Sun//Mag sensors Valid]/Kalman Gain/Create H matrix ==
  rb_hat : Inport
  bb_hat : Inport  Port=2
  3x3 0 matrix : Subsystem
  3x3 0 matrix1 : MEKF_lib/MEKF_lib/Subsystem Activated if: [All Sensors Valid] or [Gyro Bad and Sun//Mag sensors Valid]/Kalman Gain/Create H matrix/3x3 0 matrix  SystemSampleTime=-1
  Constant{1..6} (6 alike) : Constant  Value=0
  Demux1 : Demux  Outputs=3
  Demux2 : Demux  Outputs=3
  Matrix Concatenate{,1..2,5..7} (6 alike) : Concatenate  NumInputs=3  Mode=Multidimensional array  ConcatenateDimension=2
  Matrix Concatenate10 : Concatenate  Mode=Multidimensional array
  Matrix Concatenate3 : Concatenate  NumInputs=3  Mode=Multidimensional array
  Matrix Concatenate4 : Concatenate  Mode=Multidimensional array  ConcatenateDimension=2
  Matrix Concatenate8 : Concatenate  NumInputs=3  Mode=Multidimensional array
  Matrix Concatenate9 : Concatenate  Mode=Multidimensional array  ConcatenateDimension=2
  Multiply{,1..5} (6 alike) : Gain  Gain=-1
  H : Outport
  wires:
  Matrix Concatenate1/1 -> [row2rb]
  Multiply/1 -> Matrix Concatenate/2
  [mat_x] -> Matrix Concatenate4/1
  Demux1/2 -> [rb2]
  Multiply2/1 -> Matrix Concatenate2/1
  [row3rb] -> Matrix Concatenate3/3
  Matrix Concatenate/1 -> [row1rb]
  Matrix Concatenate2/1 -> [row3rb]
  [rb1] -> Multiply1/1
  [rb3] -> Multiply/1
  Multiply1/1 -> Matrix Concatenate1/3
  Constant3/1 -> Matrix Concatenate2/3
  3x3 0 matrix/1(0 3x3) -> Matrix Concatenate4/2
  [rb2] -> Multiply2/1
  [rb2] -> Matrix Concatenate/3
  [rb3] -> Matrix Concatenate1/1
  [row2rb] -> Matrix Concatenate3/2
  Constant1/1 -> Matrix Concatenate/1
  [row1rb] -> Matrix Concatenate3/1
  Demux1/1 -> [rb1]
  Matrix Concatenate3/1 -> [mat_x]
  Constant2/1 -> Matrix Concatenate1/2
  [rb1] -> Matrix Concatenate2/2
  Demux1/3 -> [rb3]
  rb_hat/1 -> Demux1/1
  Demux2/3 -> [bb3]
  bb_hat/1 -> Demux2/1
  Demux2/1 -> [bb1]
  Demux2/2 -> [bb2]
  Multiply5/1 -> Matrix Concatenate7/1
  [bb1] -> Matrix Concatenate7/2
  Constant4/1 -> Matrix Concatenate5/1
  Multiply3/1 -> Matrix Concatenate5/2
  Constant5/1 -> Matrix Concatenate6/2
  Multiply4/1 -> Matrix Concatenate6/3
  Matrix Concatenate5/1 -> [row1bb]
  [bb1] -> Multiply4/1
  Matrix Concatenate7/1 -> [row3bb]
  Constant6/1 -> Matrix Concatenate7/3
  [bb2] -> Matrix Concatenate5/3
  [bb3] -> Multiply3/1
  [bb3] -> Matrix Concatenate6/1
  [bb2] -> Multiply5/1
  Matrix Concatenate6/1 -> [row2bb]
  [row1bb] -> Matrix Concatenate8/1
  Matrix Concatenate8/1 -> [mat_xb]
  [row2bb] -> Matrix Concatenate8/2
  [row3bb] -> Matrix Concatenate8/3
  3x3 0 matrix1/1 -> Matrix Concatenate9/2
  Matrix Concatenate9/1 -> Matrix Concatenate10/2
  [mat_xb] -> Matrix Concatenate9/1
  Matrix Concatenate4/1 -> Matrix Concatenate10/1
  Matrix Concatenate10/1 -> H/1

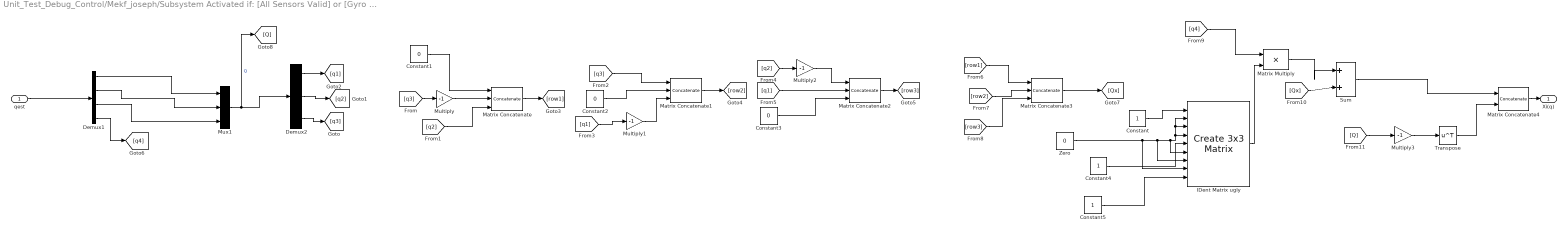
== system Unit_Test_Debug_Control/Mekf_joseph/Subsystem Activated if: [All Sensors Valid] or [Gyro Bad and Sun//Mag sensors Valid]/Kalman Gain/Makes Xi(q) Matrix ==
  qest : Inport
  Constant : Constant
  Constant1 : Constant  Value=0
  Constant2 : Constant  Value=0
  Constant3 : Constant  Value=0
  Constant4 : Constant
  Constant5 : Constant
  Demux1 : Demux
  Demux2 : Demux  Outputs=3
  IDent Matrix ugly : sharedutil/Create 3x3 Matrix  aMode=aMode
  Matrix Concatenate : Concatenate  NumInputs=3  Mode=Multidimensional array  ConcatenateDimension=2
  Matrix Concatenate1 : Concatenate  NumInputs=3  Mode=Multidimensional array  ConcatenateDimension=2
  Matrix Concatenate2 : Concatenate  NumInputs=3  Mode=Multidimensional array  ConcatenateDimension=2
  Matrix Concatenate3 : Concatenate  NumInputs=3  Mode=Multidimensional array
  Matrix Concatenate4 : Concatenate  Mode=Multidimensional array
  Matrix Multiply : Product  Inputs=**
  Multiply{,1..3} (4 alike) : Gain  Gain=-1
  Mux1 : Mux  Inputs=3
  Sum : Sum  Inputs=|++
  Transpose : Math  Operator=transpose  SaturateOnIntegerOverflow=on
  Zero : Constant  Value=0  OutDataTypeStr=Inherit: Inherit via back propagation
  Xi(q) : Outport
  wires:
  Multiply2/1 -> Matrix Concatenate2/1
  [q1] -> Matrix Concatenate2/2
  Matrix Multiply/1 -> Sum/1
  Matrix Concatenate1/1 -> [row2]
  Constant1/1 -> Matrix Concatenate/1
  Matrix Concatenate3/1 -> [Qx]
  [q2] -> Matrix Concatenate/3
  Mux1/1 -> Demux2/1, [Q]  "Q"
  Constant2/1 -> Matrix Concatenate1/2
  Demux1/2 -> Mux1/2
  [row3] -> Matrix Concatenate3/3
  qest/1 -> Demux1/1
  Multiply3/1 -> Transpose/1
  [q4] -> Matrix Multiply/1
  [q3] -> Matrix Concatenate1/1
  Demux2/2 -> [q2]
  Sum/1 -> Matrix Concatenate4/1
  [q2] -> Multiply2/1
  Demux1/4 -> [q4]
  [row2] -> Matrix Concatenate3/2
  Demux1/1 -> Mux1/1
  Demux1/3 -> Mux1/3
  Matrix Concatenate2/1 -> [row3]
  [Qx] -> Sum/2
  Multiply/1 -> Matrix Concatenate/2
  [row1] -> Matrix Concatenate3/1
  [Q] -> Multiply3/1
  Demux2/1 -> [q1]
  Transpose/1 -> Matrix Concatenate4/2
  IDent Matrix ugly/1 -> Matrix Multiply/2
  [q3] -> Multiply/1
  Matrix Concatenate/1 -> [row1]
  Demux2/3 -> [q3]
  Constant3/1 -> Matrix Concatenate2/3
  [q1] -> Multiply1/1
  Multiply1/1 -> Matrix Concatenate1/3
  Matrix Concatenate4/1 -> Xi(q)/1
  Constant/1 -> IDent Matrix ugly/1
  Constant5/1 -> IDent Matrix ugly/9
  Constant4/1 -> IDent Matrix ugly/5
  Zero/1 -> IDent Matrix ugly/8, IDent Matrix ugly/7, IDent Matrix ugly/6, IDent Matrix ugly/4, IDent Matrix ugly/3, IDent Matrix ugly/2

== system Unit_Test_Debug_Control/Mekf_joseph/Subsystem Activated if: [All Sensors Valid] or [Gyro Bad and Sun//Mag sensors Valid]/TIME PROPAGATION of Q_EST, COVARIANCE/Psi ==
  del_t : Inport
  one_half : Inport  Port=2
  om_mags : Inport  Port=3
  omega_vec : Inport  Port=4
  Divide : Product  Inputs=***
  Divide1 : Product  Inputs=**/
  Sin : Trigonometry
  "om_mags " : InportShadow  Port=3
  Psi : Outport
  wires:
  del_t/1 -> Divide/1
  Divide/1 -> Sin/1  "om_mag times0.5*del_t"
  Divide1/1 -> Psi/1  "Psi"
  om_mags/1 -> Divide/3
  Sin/1 -> Divide1/1  "sin(om_mag*0.5*del_t)"
  one_half/1 -> Divide/2
  omega_vec/1 -> Divide1/2
  "om_mags "/1 -> Divide1/3

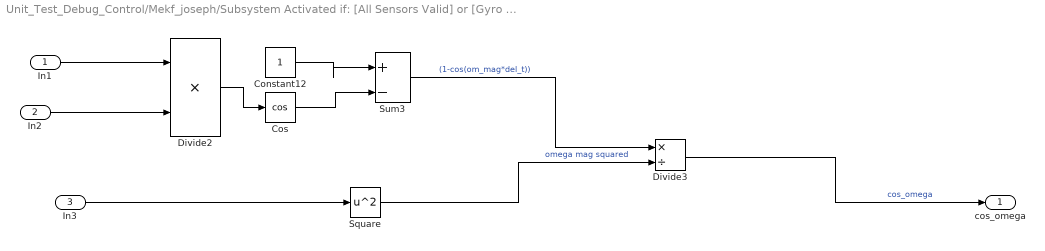
== system Unit_Test_Debug_Control/Mekf_joseph/Subsystem Activated if: [All Sensors Valid] or [Gyro Bad and Sun//Mag sensors Valid]/TIME PROPAGATION of Q_EST, COVARIANCE/cos_omega ==
  In1 : Inport
  In2 : Inport  Port=2
  In3 : Inport  Port=3
  Constant12 : Constant
  Cos : Trigonometry  Operator=cos
  Divide2 : Product  Inputs=**
  Divide3 : Product  Inputs=*/
  Square : Math  Operator=square  SaturateOnIntegerOverflow=on
  Sum3 : Sum  Inputs=|+-
  cos_omega : Outport
  wires:
  Divide2/1 -> Cos/1
  In3/1 -> Square/1
  Divide3/1 -> cos_omega/1  "cos_omega"
  Constant12/1 -> Sum3/1
  Square/1 -> Divide3/2  "omega mag squared"
  In1/1 -> Divide2/1
  Cos/1 -> Sum3/2
  In2/1 -> Divide2/2
  Sum3/1 -> Divide3/1  "(1-cos(om_mag*del_t))"

== system Unit_Test_Debug_Control/Mekf_joseph/Subsystem Activated if: [Sun//Mag Sensor Invalid and Gyros are Valid] or [Gyro Invalid and Sun//Mag sensors Invalid]/TIME PROPAGATION of Q_EST, COVARIANCE/Psi ==
  In1 : Inport
  In2 : Inport  Port=2
  om_mags : Inport  Port=3
  om_magss : Inport  Port=4
  omega_vec : Inport  Port=5
  Divide : Product  Inputs=***
  Divide1 : Product  Inputs=**/
  Sin : Trigonometry
  Psi : Outport
  wires:
  In1/1 -> Divide/1
  Divide/1 -> Sin/1  "om_mag times0.5*del_t"
  Divide1/1 -> Psi/1  "Psi"
  om_mags/1 -> Divide/3
  Sin/1 -> Divide1/1  "sin(om_mag*0.5*del_t)"
  In2/1 -> Divide/2
  omega_vec/1 -> Divide1/2
  om_magss/1 -> Divide1/3

== system Unit_Test_Debug_Control/Mekf_joseph/Subsystem Activated if: [Sun//Mag Sensor Invalid and Gyros are Valid] or [Gyro Invalid and Sun//Mag sensors Invalid]/TIME PROPAGATION of Q_EST, COVARIANCE/cos_omega ==
  In1 : Inport
  In2 : Inport  Port=2
  In3 : Inport  Port=3
  Constant12 : Constant
  Cos : Trigonometry  Operator=cos
  Divide2 : Product  Inputs=**
  Divide3 : Product  Inputs=*/
  Square : Math  Operator=square  SaturateOnIntegerOverflow=on
  Sum3 : Sum  Inputs=|+-
  cos_omega : Outport
  wires:
  Divide2/1 -> Cos/1
  In3/1 -> Square/1
  Divide3/1 -> cos_omega/1  "cos_omega"
  Constant12/1 -> Sum3/1
  Square/1 -> Divide3/2  "omega mag squared"
  In1/1 -> Divide2/1
  Cos/1 -> Sum3/2
  In2/1 -> Divide2/2
  Sum3/1 -> Divide3/1  "(1-cos(om_mag*del_t))"

== system Unit_Test_Debug_Control/Mekf_joseph/Subsystem Activated if: [All Sensors Valid] or [Gyro Bad and Sun//Mag sensors Valid]/Kalman Gain/Create H matrix/3x3 0 matrix ==
  Create 3x3 Matrix : sharedutil/Create 3x3 Matrix  aMode=aMode
  Zero : Constant  Value=0  OutDataTypeStr=Inherit: Inherit via back propagation
  0 3x3 : Outport
  wires:
  Zero/1 -> Create 3x3 Matrix/9, Create 3x3 Matrix/8, Create 3x3 Matrix/7, Create 3x3 Matrix/6, Create 3x3 Matrix/1, Create 3x3 Matrix/5, Create 3x3 Matrix/2, Create 3x3 Matrix/3, Create 3x3 Matrix/4
  Create 3x3 Matrix/1 -> 0 3x3/1

== matlab function Unit_Test_Debug_Control/Mekf_joseph/Subsystem Activated if: [Sun//Mag Sensor Invalid and Gyros are Valid] or [Gyro Invalid and Sun//Mag sensors Invalid]/TIME PROPAGATION of Q_EST, COVARIANCE/MATLAB Function ==
  data: omega_est input; om_mag output
function om_mag = om2_norm(omega_est)

om_mag = norm(omega_est);

== matlab function Unit_Test_Debug_Control/Mekf_joseph/Subsystem Activated if: [All Sensors Valid] or [Gyro Bad and Sun//Mag sensors Valid]/Kalman Gain/MATLAB Function2 ==
  data: R input; Pplus output size=[6,6]; Pminus input; H input; K output size=[6,6]
function [Pplus,K] = fcn113(R,Pminus,H)
K = Pminus*H'/(H*Pminus*H' + R);
        
        %%%Update
%         Pplus = (eye(6)-K*H)*Pminus;
        
        KHI = (K*H - eye(6));
        Pplus= KHI*Pminus*KHI' + K*R*K';
%         Pplus = (eye(6)-K*H)*Pminus*(eye(6)-K*H)' + K*R*K';
end

== matlab function Unit_Test_Debug_Control/Mekf_joseph/Subsystem Activated if: [Sun//Mag Sensor Invalid and Gyros are Valid] or [Gyro Invalid and Sun//Mag sensors Invalid]/TIME PROPAGATION of Q_EST, COVARIANCE/MATLAB Function1 ==
  data: Phi_discrete input; P_plus input; Qg input; P_prop output size=[6,6]
function P_prop = P_kplus1(Phi_discrete,P_plus,Qg)
%#codegen
P_prop = Phi_discrete*P_plus*Phi_discrete' + Qg;

== matlab function Unit_Test_Debug_Control/Mekf_joseph/Subsystem Activated if: [Sun//Mag Sensor Invalid and Gyros are Valid] or [Gyro Invalid and Sun//Mag sensors Invalid]/TIME PROPAGATION of Q_EST, COVARIANCE/MATLAB Function10 ==
  data: dt input; om_mag input; omega_x input; Phi output
function Phi = Phi_disc(dt,om_mag,omega_x)
%#codegen

% State_Trans_matrix = [(eye(3)-omega_x*sin(om_mag*del_t)/om_mag + (omega_x^2)*cos_omega),omega_x*cos_omega-eye(3)*del_t-omega_x^2*(om_mag*del_t-sin(om_mag*del_t))/om_mag^3;
%             zeros(3,3),eye(3)];

w_n     = om_mag;
w_skew  = omega_x;

% if( w_n < 1e-10 )
%     Phi = [ eye(3)     -eye(3)*dt;
%             zeros(3,3)  eye(3) ];
% else
    Phi_11  = eye(3) - w_skew*(sin(w_n*dt)/w_n) + ...
                                        w_skew^2*(1 - cos(w_n*dt))/w_n^2;
    Phi_12  = w_skew*(1 - cos(w_n*dt))/w_n^2 - eye(3)*dt - ...
                                    w_skew^2*(w_n*dt - sin(w_n*dt))/w_n^3;
    Phi_21  = zeros(3,3);    
    Phi_22  = eye(3);    
    Phi     = [ Phi_11 Phi_12;
                Phi_21 Phi_22 ];
end

== matlab function Unit_Test_Debug_Control/Mekf_joseph/Subsystem Activated if: [Sun//Mag Sensor Invalid and Gyros are Valid] or [Gyro Invalid and Sun//Mag sensors Invalid]/TIME PROPAGATION of Q_EST, COVARIANCE/MATLAB Function2 ==
  data: u input; om_mag output
function om_mag = norm_check1(u)
%#codegen
if u == 0
    om_mag = 10^-10;
else
    om_mag = u;
end
end

== matlab function Unit_Test_Debug_Control/Mekf_joseph/Subsystem Activated if: [Sun//Mag Sensor Invalid and Gyros are Valid] or [Gyro Invalid and Sun//Mag sensors Invalid]/TIME PROPAGATION of Q_EST, COVARIANCE/MATLAB Function7 ==
  data: Psi input; Psi_cross output
function Psi_cross = Psi_cross_matrix(Psi)
%#codegen

Psi_cross = [0 -Psi(3) Psi(2);
    Psi(3) 0 -Psi(1);
    -Psi(2) Psi(1) 0];


end

== matlab function Unit_Test_Debug_Control/Mekf_joseph/Subsystem Activated if: [Sun//Mag Sensor Invalid and Gyros are Valid] or [Gyro Invalid and Sun//Mag sensors Invalid]/TIME PROPAGATION of Q_EST, COVARIANCE/MATLAB Function8 ==
  data: Psi_x input; Psi input; om_mag input; del_t input; Omega_omega output
function Omega_omega = omega_omega_matrix(Psi_x,Psi,om_mag,del_t)
%#codegen

 Omega_omega = [cos(0.5*om_mag*del_t)  -Psi';
            Psi             cos(0.5*om_mag*del_t)*eye(3) - Psi_x ];

== matlab function Unit_Test_Debug_Control/Mekf_joseph/Subsystem Activated if: [Sun//Mag Sensor Invalid and Gyros are Valid] or [Gyro Invalid and Sun//Mag sensors Invalid]/TIME PROPAGATION of Q_EST, COVARIANCE/MATLAB Function9 ==
  data: omega input; omega_cross_matrix output
function omega_cross_matrix = makes_omega_cross_matrix(omega)

omega_cross_matrix = [0 -omega(3) omega(2);omega(3) 0 -omega(1);-omega(2) omega(1) 0];

== matlab function Unit_Test_Debug_Control/Mekf_joseph/Subsystem Activated if: [All Sensors Valid] or [Gyro Bad and Sun//Mag sensors Valid]/TIME PROPAGATION of Q_EST, COVARIANCE/MATLAB Function7 ==
  data: Psi input; Psi_cross output
function Psi_cross = Psi_cross_matrix(Psi)
%#codegen

Psi_cross = [0 -Psi(3) Psi(2);
    Psi(3) 0 -Psi(1);
    -Psi(2) Psi(1) 0];


end

== matlab function Unit_Test_Debug_Control/Mekf_joseph/Subsystem Activated if: [All Sensors Valid] or [Gyro Bad and Sun//Mag sensors Valid]/TIME PROPAGATION of Q_EST, COVARIANCE/MATLAB Function8 ==
  data: Psi_x input; Psi input; om_mag input; del_t input; Omega_omega output
function Omega_omega = omega_omega_matrix(Psi_x,Psi,om_mag,del_t)
%#codegen

 Omega_omega = [cos(0.5*om_mag*del_t)  -Psi';
            Psi             cos(0.5*om_mag*del_t)*eye(3) - Psi_x ];

== matlab function Unit_Test_Debug_Control/Mekf_joseph/Subsystem Activated if: [All Sensors Valid] or [Gyro Bad and Sun//Mag sensors Valid]/TIME PROPAGATION of Q_EST, COVARIANCE/MATLAB Function10 ==
  data: dt input; om_mag input; omega_x input; Phi output
function Phi = Phi_disc(dt,om_mag,omega_x)
%#codegen

% State_Trans_matrix = [(eye(3)-omega_x*sin(om_mag*del_t)/om_mag + (omega_x^2)*cos_omega),omega_x*cos_omega-eye(3)*del_t-omega_x^2*(om_mag*del_t-sin(om_mag*del_t))/om_mag^3;
%             zeros(3,3),eye(3)];

w_n     = om_mag;
w_skew  = omega_x;

% if( w_n < 1e-10 )
%     Phi = [ eye(3)     -eye(3)*dt;
%             zeros(3,3)  eye(3) ];
% else
    Phi_11  = eye(3) - w_skew*(sin(w_n*dt)/w_n) + ...
                                        w_skew*w_skew*(1 - cos(w_n*dt))/w_n^2;
    Phi_12  = w_skew*(1 - cos(w_n*dt))/w_n^2 - eye(3)*dt - ...
                                    w_skew*w_skew*(w_n*dt - sin(w_n*dt))/w_n^3;
    Phi_21  = zeros(3,3);    
    Phi_22  = eye(3);    
    Phi     = [ Phi_11 Phi_12;
                Phi_21 Phi_22 ];
end

== matlab function Unit_Test_Debug_Control/Mekf_joseph/Subsystem Activated if: [All Sensors Valid] or [Gyro Bad and Sun//Mag sensors Valid]/TIME PROPAGATION of Q_EST, COVARIANCE/MATLAB Function1 ==
  data: Phi_discrete input; P_plus input; Qg input; P_prop output size=[6,6]
function P_prop = P_kplus1(Phi_discrete,P_plus,Qg)
%#codegen
P_prop = Phi_discrete*P_plus*Phi_discrete' + Qg;

== matlab function Unit_Test_Debug_Control/Mekf_joseph/Subsystem Activated if: [All Sensors Valid] or [Gyro Bad and Sun//Mag sensors Valid]/TIME PROPAGATION of Q_EST, COVARIANCE/MATLAB Function9 ==
  data: omega input; omega_cross_matrix output
function omega_cross_matrix = makes_omega_cross_matrix(omega)

omega_cross_matrix = [0 -omega(3) omega(2);omega(3) 0 -omega(1);-omega(2) omega(1) 0];

== matlab function Unit_Test_Debug_Control/Mekf_joseph/Subsystem Activated if: [All Sensors Valid] or [Gyro Bad and Sun//Mag sensors Valid]/Kalman Gain/MATLAB Function ==
  data: qe input; XI output
function XI = fcn(qe)
%#codegen

XI = [ -qe(2) -qe(3) -qe(4);
        qe(1) -qe(4)  qe(3);
        qe(4)  qe(1) -qe(2);
       -qe(3)  qe(2)  qe(1) ];

== matlab function Unit_Test_Debug_Control/Mekf_joseph/Subsystem Activated if: [All Sensors Valid] or [Gyro Bad and Sun//Mag sensors Valid]/TIME PROPAGATION of Q_EST, COVARIANCE/MATLAB Function ==
  data: omega_est input; om_mag output
function om_mag = om2_norm(omega_est)

om_mag = norm(omega_est);

== matlab function Unit_Test_Debug_Control/Mekf_joseph/Subsystem Activated if: [All Sensors Valid] or [Gyro Bad and Sun//Mag sensors Valid]/TIME PROPAGATION of Q_EST, COVARIANCE/MATLAB Function2 ==
  data: u input; om_mag output
function om_mag = norm_check1(u)
%#codegen
if u == 0
    om_mag = 10^-10;
else
    om_mag = u;
end
end

== matlab function Unit_Test_Debug_Control/Mekf_joseph/Subsystem Activated if: [All Sensors Valid] or [Gyro Bad and Sun//Mag sensors Valid]/Kalman Gain/MATLAB Function1 ==
  data: rb_hat input; H output; bb_hat input
function H  = fcn1133(rb_hat,bb_hat)

           mat = rb_hat;
            mat_x = [0 -mat(3) mat(2);mat(3) 0 -mat(1);-mat(2) mat(1) 0]; %cross product matrix of q
        mat1 = bb_hat;
            mat_x1 = [0 -mat1(3) mat1(2);mat1(3) 0 -mat1(1);-mat1(2) mat1(1) 0];
%         Ri_x = [0 -Ri(3) Ri(2);Ri(3) 0 -Ri(1);-Ri(2) Ri(1) 0];
%         Bb_x = [0 -Bb(3) Bb(2);Bb(3) 0 -Bb(1);-Bb(2) Bb(1) 0];
%%%%% Calcualte Kalman Gain
        H = [mat_x, zeros(3,3);mat_x1,zeros(3,3)];
end

== matlab function Unit_Test_Debug_Control/Mekf_joseph/Subsystem Activated if: [All Sensors Valid] or [Gyro Bad and Sun//Mag sensors Valid]/MEASUREMENT UPDATE TO q /MATLAB Function ==
  data: qe input; qep_norm output size=[4,1]
function qep_norm = norm(qe)
%#codegen

qep_norm = 1/(norm(qe))*qe;

== matlab function Unit_Test_Debug_Control/Mekf_joseph/Subsystem Activated if: [All Sensors Valid] or [Gyro Bad and Sun//Mag sensors Valid]/Kalman Gain/MATLAB Function3 ==
  data: qe input; H output size=[6,6]; s2c_sun_eci_unit input; mag_eci_unit input; s_hat output size=[3,1]; b_hat output size=[3,1]
function [H,s_hat,b_hat] = fcn(qe,s2c_sun_eci_unit,mag_eci_unit)
%#codegen
q0 = qe(1);
qv = qe(2:4);
dcm = (2*q0^2-1)*eye(3) + 2*(qv*qv') - 2*q0*skew(qv);

s_hat = dcm*s2c_sun_eci_unit;
s_hat_x = [     0       -s_hat(3)    s_hat(2); 
             s_hat(3)       0       -s_hat(1);
            -s_hat(2)    s_hat(1)       0 ]; %cross product s_hatrix of q
        
b_hat = dcm*mag_eci_unit;
b_hat_x = [     0       -b_hat(3)    b_hat(2);
             b_hat(3)       0       -b_hat(1);
            -b_hat(2)    b_hat(1)       0 ];

H = [ s_hat_x, zeros(3,3);
      b_hat_x, zeros(3,3) ];
end
